simulink model "ask_fpga_demod"  (R2019a)
settings: Solver=VariableStepAuto  StartTime=0.0  StopTime=0.1  RelTol=1e-3
libraries: commrandsrc3 x1, dsparch4 x1
settings Model: Creator=Birkan  LastModifiedBy=Birkan

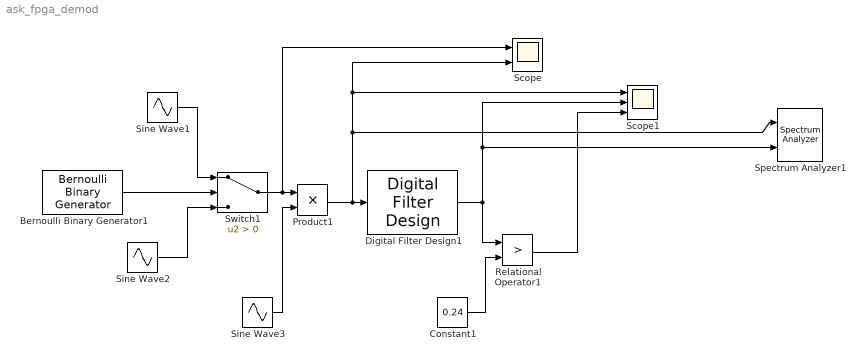
== system ask_fpga_demod ==
  Bernoulli Binary Generator1 : commrandsrc3/Bernoulli Binary Generator  ProbabilityOfZero=0.5  SeedSource=Auto  Seed=0  SampleTime=0.05  SamplesPerFrame=1  OutputDataType=double  SimulateUsing=Interpreted execution
      settings: SourceProductName=Communications Toolbox
  Constant1 : Constant  Value=0.24
  Digital Filter Design1 : dsparch4/Digital Filter Design  mwdsp_browser_bugfix_var=off
  Product1 : Product
  Relational Operator1 : RelationalOperator  Operator=>  OutDataTypeStr=boolean  RndMeth=Simplest
  Scope : Scope  NumInputPorts=2
  Scope1 : Scope  NumInputPorts=3
  Sine Wave1 : Sin  Frequency=10000*pi  SampleTime=1/1000000
  Sine Wave2 : Sin  Amplitude=0.14  Frequency=10000*pi  SampleTime=1/1000000
  Sine Wave3 : Sin  Frequency=10000*pi  SampleTime=1/1000000
  Spectrum Analyzer1 : SpectrumAnalyzer  NumInputPorts=2
  Switch1 : Switch  Criteria=u2 > Threshold
  wires:
  Constant1/1 -> Relational Operator1/2
  Relational Operator1/1 -> Scope1/3
  Switch1/1 -> Scope/1, Product1/1
  Bernoulli Binary Generator1/1 -> Switch1/2
  Sine Wave3/1 -> Product1/2
  Sine Wave2/1 -> Switch1/3
  Digital Filter Design1/1 -> Scope1/2, Spectrum Analyzer1/2, Relational Operator1/1
  Sine Wave1/1 -> Switch1/1
  Product1/1 -> Scope/2, Scope1/1, Spectrum Analyzer1/1, Digital Filter Design1/1
